simulink model "BMS_CurrentLimitsCalc_COM"  (R2022b)
settings: configuration reference "BMS_Sw_CodeGenConfig" (kept outside this file)
model workspace: external: MAT-File H:\0\New MAAM\10 - MBD\Battary Management System\SWE.3 CDD\DataTypes\Data_Script.mat (data not in the file)
undefined symbols (not defined in the file): BATT, Schedule
libraries: simulink x1
settings Model: DataDictionary=BMS_Arch_DD.sldd  Creator=MAAM  LastModifiedBy=MAAM
settings ConfigSetRef: SourceName=BMS_Sw_CodeGenConfig

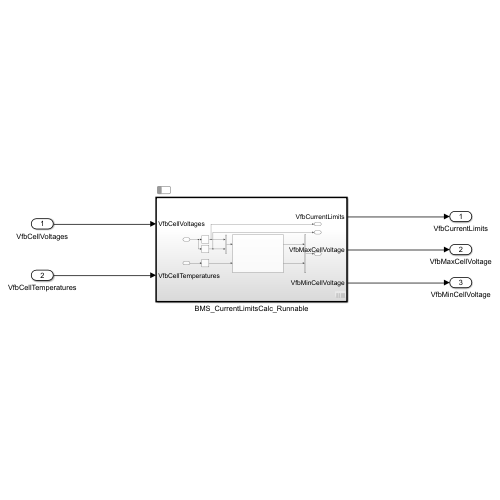
[thumbnail: Simulink's stored preview of the top-level diagram]
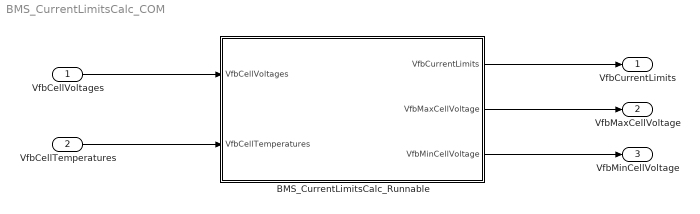
== system BMS_CurrentLimitsCalc_COM ==
  VfbCellVoltages : Inport  OutDataTypeStr=single  Unit=V  PortDimensions=BATT.Package.NumModules
  VfbCellTemperatures : Inport  Port=2  OutDataTypeStr=single  Unit=°C  PortDimensions=BATT.Package.NumModules
  BMS_CurrentLimitsCalc_Runnable : Subsystem  Tag=BMS_CurrentLimitsCalc_Task  Priority=0  TreatAsAtomicUnit=on  ScheduleAs=Periodic partition  PartitionName=BMS_CurrentLimitsCalc_Task  SystemSampleTime=Schedule.BMS_CurrentLimitsCalc_Task  RTWFileName=BMS_CULM_COM
      settings: RTWSystemCode=Nonreusable function  RTWFcnNameOpts=Use subsystem name  FunctionInterfaceSpec=Allow arguments (Optimized)
  VfbCurrentLimits : Outport  OutDataTypeStr=single  Unit=A
  VfbMaxCellVoltage : Outport  Port=2  OutDataTypeStr=single  Unit=V  PortDimensions=1
  VfbMinCellVoltage : Outport  Port=3  OutDataTypeStr=single  Unit=V  PortDimensions=1
  wires:
  BMS_CurrentLimitsCalc_Runnable/1(VfbCurrentLimits) -> VfbCurrentLimits/1
  BMS_CurrentLimitsCalc_Runnable/2(VfbMaxCellVoltage) -> VfbMaxCellVoltage/1
  BMS_CurrentLimitsCalc_Runnable/3(VfbMinCellVoltage) -> VfbMinCellVoltage/1
  VfbCellTemperatures/1 -> BMS_CurrentLimitsCalc_Runnable/2(VfbCellTemperatures)
  VfbCellVoltages/1 -> BMS_CurrentLimitsCalc_Runnable/1(VfbCellVoltages)

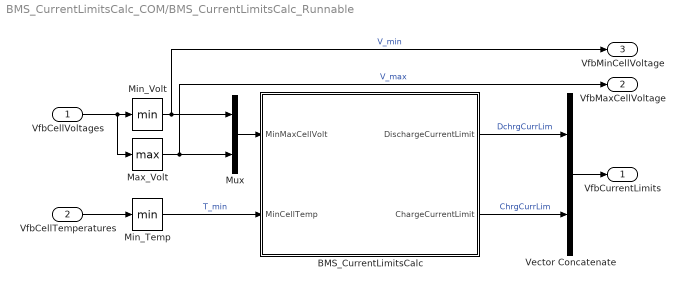
== system BMS_CurrentLimitsCalc_COM/BMS_CurrentLimitsCalc_Runnable ==
  VfbCellVoltages : Inport
  VfbCellTemperatures : Inport  Port=2
  BMS_CurrentLimitsCalc : Subsystem
  Max_Volt : MinMax  Function=max  InputSameDT=on  OutDataTypeStr=single
  Min_Temp : MinMax  InputSameDT=on  OutDataTypeStr=single
  Min_Volt : MinMax  InputSameDT=on  OutDataTypeStr=single
  Mux : Mux  Inputs=2
  Vector Concatenate : Concatenate
  VfbCurrentLimits : Outport
  VfbMaxCellVoltage : Outport  Port=2
  VfbMinCellVoltage : Outport  Port=3
  wires:
  BMS_CurrentLimitsCalc/2(ChargeCurrentLimit) -> Vector Concatenate/2  "ChrgCurrLim"
  BMS_CurrentLimitsCalc/1(DischargeCurrentLimit) -> Vector Concatenate/1  "DchrgCurrLim"
  Min_Volt/1 -> Mux/1, VfbMinCellVoltage/1  "V_min"
  Max_Volt/1 -> Mux/2, VfbMaxCellVoltage/1  "V_max"
  Vector Concatenate/1 -> VfbCurrentLimits/1
  VfbCellVoltages/1 -> Max_Volt/1, Min_Volt/1
  Mux/1 -> BMS_CurrentLimitsCalc/1(MinMaxCellVolt)
  VfbCellTemperatures/1 -> Min_Temp/1
  Min_Temp/1 -> BMS_CurrentLimitsCalc/2(MinCellTemp)  "T_min"

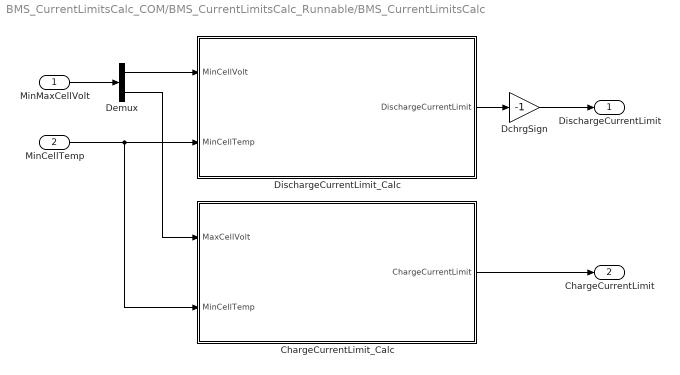
== system BMS_CurrentLimitsCalc_COM/BMS_CurrentLimitsCalc_Runnable/BMS_CurrentLimitsCalc ==
  MinMaxCellVolt : Inport
  MinCellTemp : Inport  Port=2
  ChargeCurrentLimit_Calc : Subsystem  TreatAsAtomicUnit=on
      settings: RTWSystemCode=Nonreusable function  RTWFcnNameOpts=Use subsystem name  FunctionInterfaceSpec=Allow arguments (Optimized)
  DchrgSign : Gain  Gain=-1
  Demux : Demux  Outputs=2
  DischargeCurrentLimit_Calc : Subsystem  TreatAsAtomicUnit=on
      settings: RTWSystemCode=Nonreusable function  RTWFcnNameOpts=Use subsystem name  FunctionInterfaceSpec=Allow arguments (Optimized)
  DischargeCurrentLimit : Outport
  ChargeCurrentLimit : Outport  Port=2
  wires:
  ChargeCurrentLimit_Calc/1(ChargeCurrentLimit) -> ChargeCurrentLimit/1
  DischargeCurrentLimit_Calc/1(DischargeCurrentLimit) -> DchrgSign/1
  MinMaxCellVolt/1 -> Demux/1
  Demux/1 -> DischargeCurrentLimit_Calc/1(MinCellVolt)
  Demux/2 -> ChargeCurrentLimit_Calc/1(MaxCellVolt)
  MinCellTemp/1 -> ChargeCurrentLimit_Calc/2(MinCellTemp), DischargeCurrentLimit_Calc/2(MinCellTemp)
  DchrgSign/1 -> DischargeCurrentLimit/1

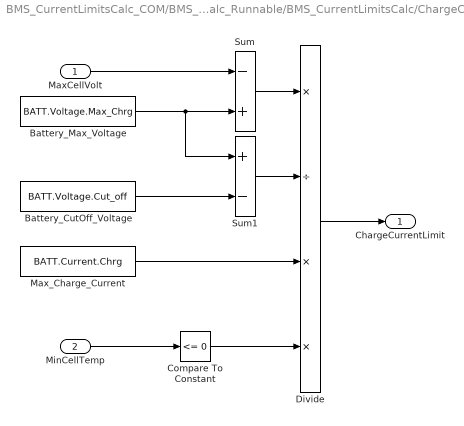
== system BMS_CurrentLimitsCalc_COM/BMS_CurrentLimitsCalc_Runnable/BMS_CurrentLimitsCalc/ChargeCurrentLimit_Calc ==
  MaxCellVolt : Inport
  MinCellTemp : Inport  Port=2
  Battery_CutOff_Voltage : Constant  Value=BATT.Voltage.Cut_off  OutDataTypeStr=single
  Battery_Max_Voltage : Constant  Value=BATT.Voltage.Max_Chrg  OutDataTypeStr=single
  Compare To Constant : simulink/Logic and Bit Operations/Compare To Constant  relop=<=  const=0  OutDataTypeStr=uint8
  Divide : Product  Inputs=*/**
  Max_Charge_Current : Constant  Value=BATT.Current.Chrg  OutDataTypeStr=single
  Sum : Sum  Inputs=-+
  Sum1 : Sum  Inputs=+-
  ChargeCurrentLimit : Outport
  wires:
  MinCellTemp/1 -> Compare To Constant/1
  Sum/1 -> Divide/1
  Sum1/1 -> Divide/2
  Max_Charge_Current/1 -> Divide/3
  MaxCellVolt/1 -> Sum/1
  Battery_Max_Voltage/1 -> Sum1/1, Sum/2
  Divide/1 -> ChargeCurrentLimit/1
  Compare To Constant/1 -> Divide/4
  Battery_CutOff_Voltage/1 -> Sum1/2

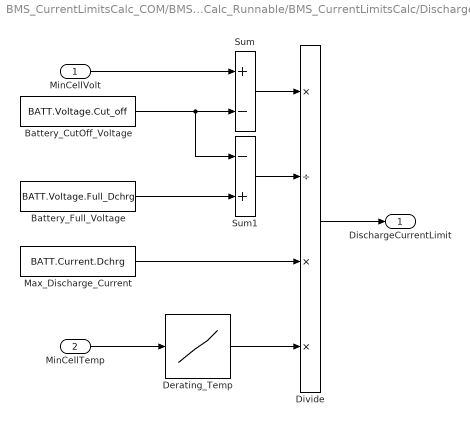
== system BMS_CurrentLimitsCalc_COM/BMS_CurrentLimitsCalc_Runnable/BMS_CurrentLimitsCalc/DischargeCurrentLimit_Calc ==
  MinCellVolt : Inport
  MinCellTemp : Inport  Port=2
  Battery_CutOff_Voltage : Constant  Value=BATT.Voltage.Cut_off  OutDataTypeStr=single
  Battery_Full_Voltage : Constant  Value=BATT.Voltage.Full_Dchrg  OutDataTypeStr=single
  Derating_Temp : Lookup_n-D  NumberOfTableDimensions=1  BreakpointsForDimension1=BATT.Temperature.T_LUT  Table=BATT.Temperature.derate_Fact  InternalRulePriority=Speed  RndMeth=Simplest
  Divide : Product  Inputs=*/**
  Max_Discharge_Current : Constant  Value=BATT.Current.Dchrg  OutDataTypeStr=single
  Sum : Sum  Inputs=+-
  Sum1 : Sum  Inputs=-+
  DischargeCurrentLimit : Outport
  wires:
  MinCellTemp/1 -> Derating_Temp/1
  Derating_Temp/1 -> Divide/4
  Max_Discharge_Current/1 -> Divide/3
  Divide/1 -> DischargeCurrentLimit/1
  Sum/1 -> Divide/1
  Sum1/1 -> Divide/2
  MinCellVolt/1 -> Sum/1
  Battery_CutOff_Voltage/1 -> Sum1/1, Sum/2
  Battery_Full_Voltage/1 -> Sum1/2
